simulink model "FDIBenchMark_BLW_66_71"  (Simulink 6.3)
settings: Solver=ode45  StartTime=0.0  StopTime=300  FixedStep=Ts  RelTol=1e-12
InitFcn:
  | FDIBenchMarkData
undefined symbols (not defined in the file or in its folder): a, Addt, Addt2, alpha, alpha_gc, Apb, Apb1, Apb2, Bddt, Bddt2, Bpb, Bpb1, Bpb2, Cddt, Constant_Beta_1_m1, Constant_Beta_3_m1, Constant_Omega_r_m1, Constant_tau_gc, Cpb, Cpb1, Cpb2, Cq, DiscIntNeverNeededParam, eta_gc, Gain_Beta_2_m2, Gain_Omega_r_m2, H, k, K_i, K_opt, K_p, L, m, m_vw, Omega_delta, omega_n, Omega_nom, P_r, R, r, r0, rho, seed, T_sample, Ts, turb_int, turbulence_seeds, u0, xi
libraries: simulink x13
settings Model: Creator=peodg  LastModifiedBy=Administrator  StrictBusMsg=None
settings DebuggingCC: SignalResolutionControl=UseLocalSettings  MultiTaskDSMMsg=error
settings HardwareCC: TargetHWDeviceType=32-bit Generic

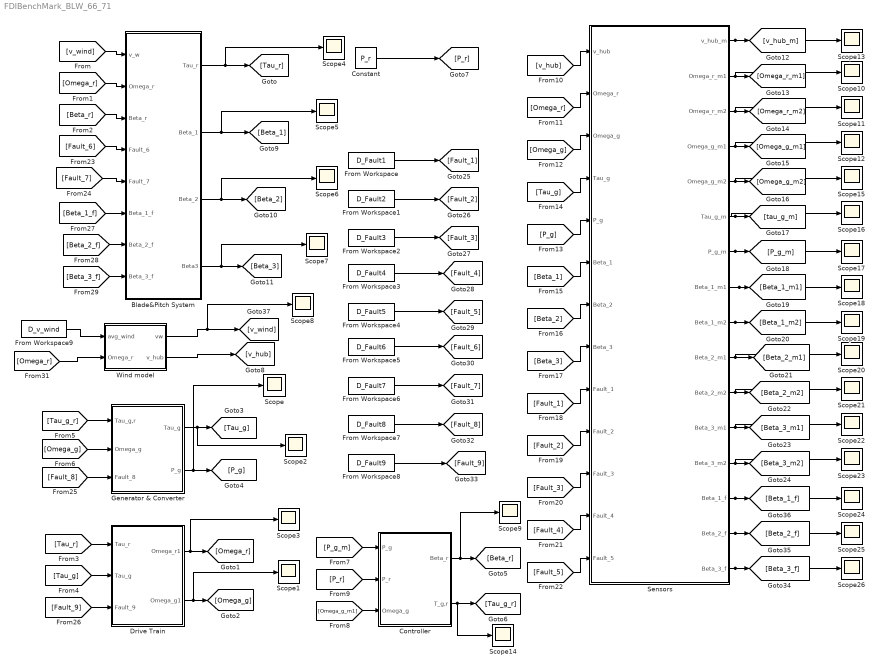
== system FDIBenchMark_BLW_66_71 ==
  Blade&Pitch System : Subsystem
  Constant : Constant  Value=P_r
  Controller : Subsystem
  Drive Train : Subsystem
  From Workspace : FromWorkspace  VariableName=D_Fault1  SampleTime=Ts
  From Workspace1 : FromWorkspace  VariableName=D_Fault2  SampleTime=Ts
  From Workspace2 : FromWorkspace  VariableName=D_Fault3  SampleTime=Ts
  From Workspace3 : FromWorkspace  VariableName=D_Fault4  SampleTime=Ts
  From Workspace4 : FromWorkspace  VariableName=D_Fault5  SampleTime=Ts
  From Workspace5 : FromWorkspace  VariableName=D_Fault6  SampleTime=Ts
  From Workspace6 : FromWorkspace  VariableName=D_Fault7  SampleTime=Ts
  From Workspace7 : FromWorkspace  VariableName=D_Fault8  SampleTime=Ts
  From Workspace8 : FromWorkspace  VariableName=D_Fault9  SampleTime=Ts
  From Workspace9 : FromWorkspace  VariableName=D_v_wind
  Generator & Converter : Subsystem
  Scope{,1..26} (27 alike) : Scope
      Scope settings: YMin=1e+006  YMax=5.25e+006  SaveName=P_g  DataFormat=Array  SampleInput=on  SampleTime=Ts
      Scope1 settings: YMin=64  YMax=66.25  SaveName=Oemga_g1  DataFormat=Array  SampleInput=on  SampleTime=Ts
      Scope10 settings: YMin=1.1  YMax=2.4  SaveName=Omega_r_m1  DataFormat=Array  SampleInput=on  SampleTime=Ts
      Scope11 settings: YMin=-1  YMax=1  SaveName=Omega_r_m2  DataFormat=Array  SampleInput=on  SampleTime=Ts
      Scope12 settings: YMin=-1  YMax=1  SaveName=Omega_g_m1  DataFormat=Array  SampleInput=on  SampleTime=Ts
      Scope13 settings: YMin=-1  YMax=1  SaveName=v_hub_m  DataFormat=Array  SampleInput=on  SampleTime=Ts
      Scope14 settings: YMin=-2.5  YMax=20  SaveName=T_g_r  DataFormat=Array  SampleInput=on  SampleTime=Ts
      Scope15 settings: YMin=-1  YMax=1  SaveName=Omega_g_m2  DataFormat=Array  SampleInput=on  SampleTime=Ts
      Scope16 settings: YMin=-1  YMax=1  SaveName=Tau_g_m  DataFormat=Array  SampleInput=on  SampleTime=Ts
      Scope17 settings: YMin=-1  YMax=1  SaveName=P_g_m  DataFormat=Array  SampleInput=on  SampleTime=Ts
      Scope18 settings: YMin=-1  YMax=1  SaveName=Beta_1_m1  DataFormat=Array  SampleInput=on  SampleTime=Ts
      Scope19 settings: YMin=-1  YMax=1  SaveName=Beta_1_m2  DataFormat=Array  SampleInput=on  SampleTime=Ts
      Scope2 settings: YMin=29400  YMax=29875  SaveName=Tau_g  DataFormat=Array  SampleInput=on  SampleTime=Ts
      Scope20 settings: YMin=-1  YMax=1  SaveName=Beta_2_m1  DataFormat=Array  SampleInput=on  SampleTime=Ts
      Scope21 settings: YMin=-1  YMax=1  SaveName=Beta_2_m2  DataFormat=Array  SampleInput=on  SampleTime=Ts
      Scope22 settings: YMin=-4  YMax=12  SaveName=Beta_3_m1  DataFormat=Array  SampleInput=on  SampleTime=Ts
      Scope23 settings: YMin=-1  YMax=1  SaveName=Beta_3_m2  DataFormat=Array  SampleInput=on  SampleTime=Ts
      Scope24 settings: YMin=-1  YMax=1  SaveName=Beta_1_f  DataFormat=Array  SampleInput=on  SampleTime=Ts
      Scope25 settings: YMin=-1  YMax=1  SaveName=Beta_2_f  DataFormat=Array  SampleInput=on  SampleTime=Ts
      Scope26 settings: YMin=-1  YMax=1  SaveName=Beta_3_f  DataFormat=Array  SampleInput=on  SampleTime=Ts
      Scope3 settings: YMin=0.62  YMax=0.69  SaveName=Omega_r1  DataFormat=Array  SampleInput=on  SampleTime=Ts
      Scope4 settings: YMin=-1e+006  YMax=6e+006  SaveName=Tau_r  DataFormat=Array  SampleInput=on  SampleTime=Ts
      Scope5 settings: YMin=-3  YMax=8  SaveName=Beta1  DataFormat=Array  SampleInput=on  SampleTime=Ts
      Scope6 settings: YMin=-0.3  YMax=0.3  SaveName=Beta  DataFormat=Array  SampleInput=on  SampleTime=Ts
      Scope7 settings: YMin=-2.5  YMax=3.5  SaveName=Beta3  DataFormat=Array  SampleInput=on  SampleTime=Ts
      Scope8 settings: YMin=3  YMax=18  SaveName=Vw  DataFormat=Array  SampleInput=on  SampleTime=Ts
      Scope9 settings: YMin=-2.5  YMax=20  SaveName=Beta_r  DataFormat=Array  SampleInput=on  SampleTime=Ts
  Sensors : Subsystem
  Wind model : Subsystem
  wires:
  [v_wind] -> Blade&Pitch System/1(v_w)
  [Omega_r] -> Blade&Pitch System/2(Omega_r)
  [Beta_r] -> Blade&Pitch System/3(Beta_r)
  [Tau_r] -> Drive Train/1(Tau_r)
  [Tau_g] -> Drive Train/2(Tau_g)
  Drive Train/1(Omega_r1) -> [Omega_r], Scope3/1
  [Tau_g_r] -> Generator & Converter/1(Tau_g,r)
  [Omega_g] -> Generator & Converter/2(Omega_g)
  Generator & Converter/1(Tau_g) -> [Tau_g], Scope2/1
  Generator & Converter/2(P_g) -> [P_g], Scope/1
  [P_g_m] -> Controller/1(P_g)
  [Omega_g_m1] -> Controller/3(Omega_g)
  Controller/1(Beta_r) -> [Beta_r], Scope9/1
  Controller/2(T_g,r) -> [Tau_g_r], Scope14/1
  [P_r] -> Controller/2(P_r)
  Constant/1 -> [P_r]
  Sensors/1(v_hub_m) -> [v_hub_m], Scope13/1
  Sensors/2(Omega_r_m1) -> [Omega_r_m1], Scope10/1
  Sensors/3(Omega_r_m2) -> [Omega_r_m2], Scope11/1
  Sensors/4(Omega_g_m1) -> [Omega_g_m1], Scope12/1
  Sensors/5(Omega_g_m2) -> [Omega_g_m2], Scope15/1
  Sensors/6(Tau_g_m) -> [tau_g_m], Scope16/1
  Sensors/7(P_g_m) -> [P_g_m], Scope17/1
  Sensors/8(Beta_1_m1) -> [Beta_1_m1], Scope18/1
  Sensors/9(Beta_1_m2) -> [Beta_1_m2], Scope19/1
  Sensors/10(Beta_2_m1) -> [Beta_2_m1], Scope20/1
  Sensors/11(Beta_2_m2) -> [Beta_2_m2], Scope21/1
  Sensors/12(Beta_3_m1) -> [Beta_3_m1], Scope22/1
  Sensors/13(Beta_3_m2) -> [Beta_3_m2], Scope23/1
  [v_hub] -> Sensors/1(v_hub)
  [Omega_r] -> Sensors/2(Omega_r)
  [Omega_g] -> Sensors/3(Omega_g)
  [Tau_g] -> Sensors/4(Tau_g)
  [P_g] -> Sensors/5(P_g)
  [Beta_1] -> Sensors/6(Beta_1)
  [Beta_2] -> Sensors/7(Beta_2)
  [Beta_3] -> Sensors/8(Beta_3)
  [Fault_1] -> Sensors/9(Fault_1)
  [Fault_2] -> Sensors/10(Fault_2)
  [Fault_3] -> Sensors/11(Fault_3)
  [Fault_4] -> Sensors/12(Fault_4)
  [Fault_5] -> Sensors/13(Fault_5)
  [Fault_6] -> Blade&Pitch System/4(Fault_6)
  [Fault_7] -> Blade&Pitch System/5(Fault_7)
  [Fault_8] -> Generator & Converter/3(Fault_8)
  [Fault_9] -> Drive Train/3(Fault_9)
  From Workspace8/1 -> [Fault_9]
  From Workspace7/1 -> [Fault_8]
  From Workspace6/1 -> [Fault_7]
  From Workspace5/1 -> [Fault_6]
  From Workspace4/1 -> [Fault_5]
  From Workspace3/1 -> [Fault_4]
  From Workspace2/1 -> [Fault_3]
  From Workspace1/1 -> [Fault_2]
  From Workspace/1 -> [Fault_1]
  Drive Train/2(Omega_g1) -> [Omega_g], Scope1/1
  Sensors/16(Beta_3_f) -> [Beta_3_f], Scope26/1
  Sensors/15(Beta_2_f) -> [Beta_2_f], Scope25/1
  Sensors/14(Beta_1_f) -> [Beta_1_f], Scope24/1
  [Beta_1_f] -> Blade&Pitch System/6(Beta_1_f)
  [Beta_2_f] -> Blade&Pitch System/7(Beta_2_f)
  [Beta_3_f] -> Blade&Pitch System/8(Beta_3_f)
  Blade&Pitch System/4(Beta3) -> [Beta_3], Scope7/1
  Blade&Pitch System/3(Beta_2) -> [Beta_2], Scope6/1
  Blade&Pitch System/2(Beta_1) -> [Beta_1], Scope5/1
  Blade&Pitch System/1(Tau_r) -> [Tau_r], Scope4/1
  Wind model/1(vw) -> [v_wind], Scope8/1
  Wind model/2(v_hub) -> [v_hub]
  [Omega_r] -> Wind model/2(Omega_r)
  From Workspace9/1 -> Wind model/1(avg_wind)

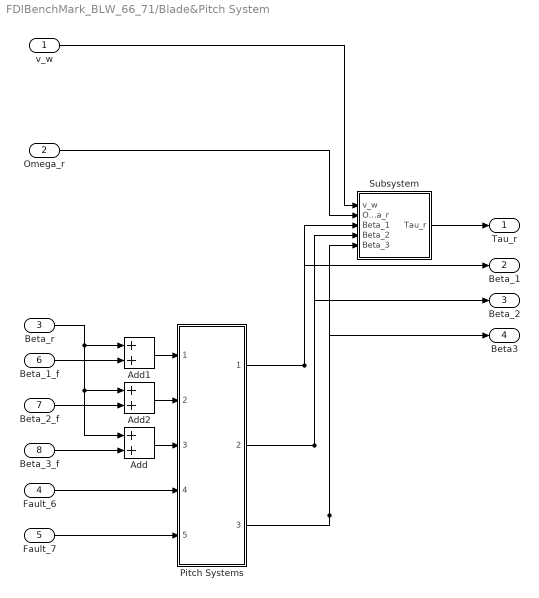
== system FDIBenchMark_BLW_66_71/Blade&Pitch System ==
  v_w : Inport
  Omega_r : Inport  Port=2
  Beta_r : Inport  Port=3
  Fault_6 : Inport  Port=4
  Fault_7 : Inport  Port=5
  Beta_1_f : Inport  Port=6
  Beta_2_f : Inport  Port=7
  Beta_3_f : Inport  Port=8
  Add : Sum  OutScaling=2^-10
  Add1 : Sum  OutScaling=2^-10
  Add2 : Sum  OutScaling=2^-10
  Pitch Systems : Subsystem
  Subsystem : Subsystem
  Tau_r : Outport
  Beta_1 : Outport  Port=2
  Beta_2 : Outport  Port=3
  Beta3 : Outport  Port=4
  wires:
  Pitch Systems/1(Beta_1) -> Subsystem/3(Beta_1), Beta_1/1
  Pitch Systems/2(Beta_2) -> Subsystem/4(Beta_2), Beta_2/1
  Pitch Systems/3(Beta_3) -> Subsystem/5(Beta_3), Beta3/1
  Subsystem/1(Tau_r) -> Tau_r/1
  v_w/1 -> Subsystem/1(v_w)
  Omega_r/1 -> Subsystem/2(Omega_r)
  Fault_6/1 -> Pitch Systems/4(Fault_6)
  Fault_7/1 -> Pitch Systems/5(Fault_7)
  Add/1 -> Pitch Systems/3(Beta_r3)
  Add1/1 -> Pitch Systems/1(Beta_r1)
  Add2/1 -> Pitch Systems/2(Beta_r2)
  Beta_3_f/1 -> Add/2
  Beta_2_f/1 -> Add2/2
  Beta_1_f/1 -> Add1/2
  Beta_r/1 -> Add1/1, Add2/1, Add/1

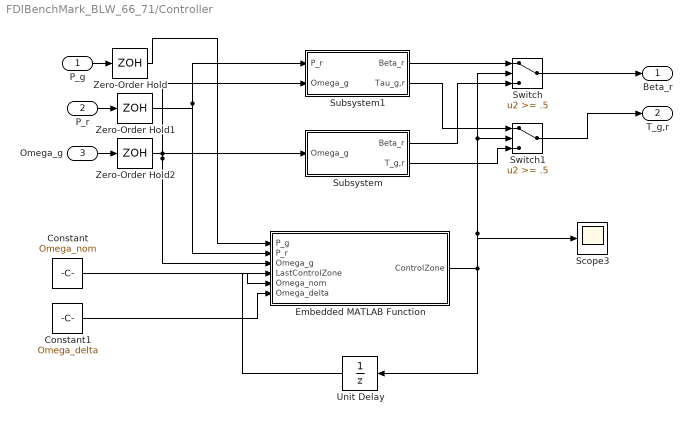
== system FDIBenchMark_BLW_66_71/Controller ==
  P_g : Inport
  P_r : Inport  Port=2
  Omega_g : Inport  Port=3
  Constant : Constant  Value=Omega_nom
  Constant1 : Constant  Value=Omega_delta
  Embedded MATLAB Function : Stateflow chart  TreatAsAtomicUnit=on
      settings: PermitHierarchicalResolution=ParametersOnly
  Scope3 : Scope
      settings: YMin=0.62  YMax=0.69  SaveName=Omega_r  DataFormat=Array  SampleInput=on  SampleTime=Ts
  Subsystem : Subsystem
  Subsystem1 : Subsystem
  Switch : Switch  Threshold=.5
  Switch1 : Switch  Threshold=.5
  Unit Delay : UnitDelay  Orientation=left  SampleTime=Ts
  Zero-Order Hold : ZeroOrderHold  SampleTime=Ts
  Zero-Order Hold1 : ZeroOrderHold  SampleTime=Ts
  Zero-Order Hold2 : ZeroOrderHold  SampleTime=Ts
  Beta_r : Outport
  T_g,r : Outport  Port=2
  wires:
  Embedded MATLAB Function/1(ControlZone) -> Unit Delay/1, Switch/2, Switch1/2, Scope3/1
  Unit Delay/1 -> Embedded MATLAB Function/4(LastControlZone)
  P_g/1 -> Zero-Order Hold/1
  P_r/1 -> Zero-Order Hold1/1
  Omega_g/1 -> Zero-Order Hold2/1
  Switch/1 -> Beta_r/1
  Switch1/1 -> T_g,r/1
  Subsystem1/1(Beta_r) -> Switch/1
  Subsystem/1(Beta_r) -> Switch/3
  Subsystem1/2(Tau_g,r) -> Switch1/1
  Subsystem/2(T_g,r) -> Switch1/3
  Constant/1 -> Embedded MATLAB Function/5(Omega_nom)
  Constant1/1 -> Embedded MATLAB Function/6(Omega_delta)
  Zero-Order Hold/1 -> Embedded MATLAB Function/1(P_g)
  Zero-Order Hold1/1 -> Embedded MATLAB Function/2(P_r), Subsystem1/1(P_r)
  Zero-Order Hold2/1 -> Embedded MATLAB Function/3(Omega_g), Subsystem1/2(Omega_g), Subsystem/1(Omega_g)

== system FDIBenchMark_BLW_66_71/Drive Train ==
  Tau_r : Inport
  Tau_g : Inport  Port=2
  Fault_9 : Inport  Port=3
  Add : Sum  OutScaling=2^-10
  Demux1 : Demux  Outputs=2
  Gain : Gain  Orientation=left  Gain=Addt  Multiplication=Matrix(K*u)
  Gain1 : Gain  Gain=Bddt  Multiplication=Matrix(K*u)
  Gain2 : Gain  Gain=Cddt  Multiplication=Matrix(K*u)
  Gain3 : Gain  Orientation=left  Gain=Addt2  Multiplication=Matrix(K*u)
  Gain4 : Gain  Gain=Bddt2  Multiplication=Matrix(K*u)
  Integrator : Integrator  InitialCondition=[1 100 0]
  Mux : Mux  Inputs=2
  Switch1 : Switch  Threshold=0.5
  Switch2 : Switch  Orientation=left  Threshold=0.5
  Omega_r1 : Outport
  Omega_g1 : Outport  Port=2
  wires:
  Tau_r/1 -> Mux/1
  Tau_g/1 -> Mux/2
  Integrator/1 -> Gain2/1, Gain/1, Gain3/1
  Add/1 -> Integrator/1
  Switch1/1 -> Add/1
  Gain1/1 -> Switch1/1
  Gain4/1 -> Switch1/3
  Gain/1 -> Switch2/1
  Gain3/1 -> Switch2/3
  Switch2/1 -> Add/2
  Demux1/1 -> Omega_r1/1
  Demux1/2 -> Omega_g1/1
  Gain2/1 -> Demux1/1
  Fault_9/1 -> Switch1/2, Switch2/2
  Mux/1 -> Gain1/1, Gain4/1

== system FDIBenchMark_BLW_66_71/Generator & Converter ==
  Tau_g,r : Inport
  Omega_g : Inport  Port=2
  Fault_8 : Inport  Port=3
  Bias : Bias  Bias=Constant_tau_gc
  Divide : Product  Inputs=**  OutScaling=2^-10
  Gain : Gain  Gain=eta_gc
  Switch : Switch  Threshold=0.5
  Transfer Fcn : TransferFcn  Numerator=[alpha_gc]  Denominator=[1 alpha_gc]
  Tau_g : Outport
  P_g : Outport  Port=2
  wires:
  Tau_g,r/1 -> Transfer Fcn/1
  Gain/1 -> P_g/1
  Divide/1 -> Gain/1
  Omega_g/1 -> Divide/2
  Transfer Fcn/1 -> Bias/1, Switch/1
  Fault_8/1 -> Switch/2
  Switch/1 -> Divide/1, Tau_g/1
  Bias/1 -> Switch/3

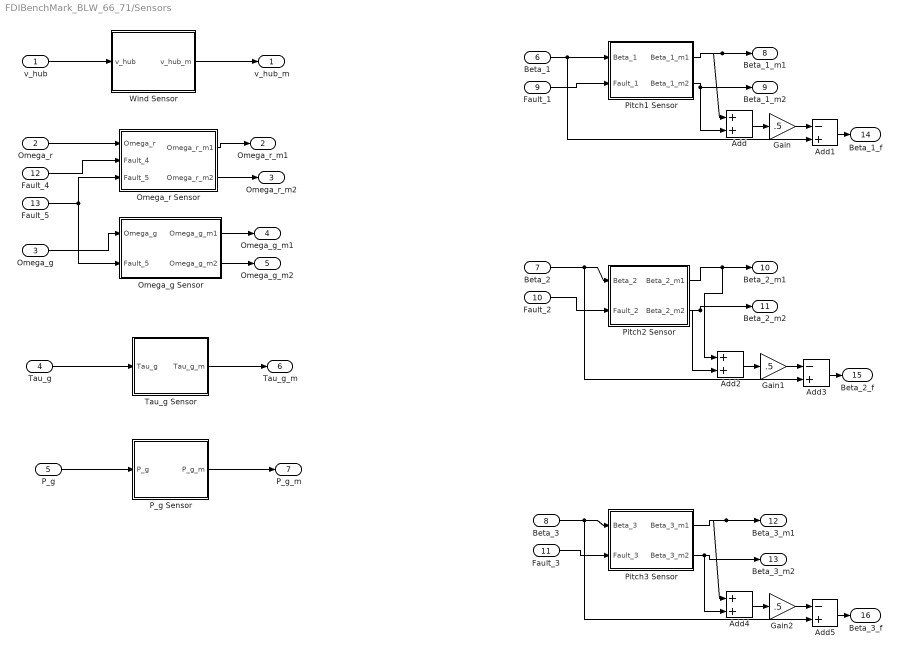
== system FDIBenchMark_BLW_66_71/Sensors ==
  v_hub : Inport
  Omega_r : Inport  Port=2
  Omega_g : Inport  Port=3
  Tau_g : Inport  Port=4
  P_g : Inport  Port=5
  Beta_1 : Inport  Port=6
  Beta_2 : Inport  Port=7
  Beta_3 : Inport  Port=8
  Fault_1 : Inport  Port=9
  Fault_2 : Inport  Port=10
  Fault_3 : Inport  Port=11
  Fault_4 : Inport  Port=12
  Fault_5 : Inport  Port=13
  Add : Sum  OutScaling=2^-10
  Add1 : Sum  Inputs=-+  OutScaling=2^-10
  Add2 : Sum  OutScaling=2^-10
  Add3 : Sum  Inputs=-+  OutScaling=2^-10
  Add4 : Sum  OutScaling=2^-10
  Add5 : Sum  Inputs=-+  OutScaling=2^-10
  Gain : Gain  Gain=.5
  Gain1 : Gain  Gain=.5
  Gain2 : Gain  Gain=.5
  Omega_g Sensor : Subsystem
  Omega_r Sensor : Subsystem
  P_g Sensor : Subsystem
  Pitch1 Sensor : Subsystem
  Pitch2 Sensor : Subsystem
  Pitch3 Sensor : Subsystem
  Tau_g Sensor : Subsystem
  Wind Sensor : Subsystem
  v_hub_m : Outport
  Omega_r_m1 : Outport  Port=2
  Omega_r_m2 : Outport  Port=3
  Omega_g_m1 : Outport  Port=4
  Omega_g_m2 : Outport  Port=5
  Tau_g_m : Outport  Port=6
  P_g_m : Outport  Port=7
  Beta_1_m1 : Outport  Port=8
  Beta_1_m2 : Outport  Port=9
  Beta_2_m1 : Outport  Port=10
  Beta_2_m2 : Outport  Port=11
  Beta_3_m1 : Outport  Port=12
  Beta_3_m2 : Outport  Port=13
  Beta_1_f : Outport  Port=14
  Beta_2_f : Outport  Port=15
  Beta_3_f : Outport  Port=16
  wires:
  Wind Sensor/1(v_hub_m) -> v_hub_m/1
  v_hub/1 -> Wind Sensor/1(v_hub)
  Omega_r/1 -> Omega_r Sensor/1(Omega_r)
  Omega_r Sensor/1(Omega_r_m1) -> Omega_r_m1/1
  Omega_r Sensor/2(Omega_r_m2) -> Omega_r_m2/1
  Omega_g/1 -> Omega_g Sensor/1(Omega_g)
  Omega_g Sensor/1(Omega_g_m1) -> Omega_g_m1/1
  Omega_g Sensor/2(Omega_g_m2) -> Omega_g_m2/1
  Tau_g/1 -> Tau_g Sensor/1(Tau_g)
  Tau_g Sensor/1(Tau_g_m) -> Tau_g_m/1
  P_g/1 -> P_g Sensor/1(P_g)
  P_g Sensor/1(P_g_m) -> P_g_m/1
  Beta_1/1 -> Pitch1 Sensor/1(Beta_1), Add1/2
  Pitch1 Sensor/1(Beta_1_m1) -> Beta_1_m1/1, Add/1
  Pitch1 Sensor/2(Beta_1_m2) -> Beta_1_m2/1, Add/2
  Beta_2/1 -> Pitch2 Sensor/1(Beta_2), Add3/2
  Pitch2 Sensor/1(Beta_2_m1) -> Beta_2_m1/1, Add2/1
  Pitch2 Sensor/2(Beta_2_m2) -> Beta_2_m2/1, Add2/2
  Beta_3/1 -> Pitch3 Sensor/1(Beta_3), Add5/2
  Pitch3 Sensor/1(Beta_3_m1) -> Beta_3_m1/1, Add4/1
  Pitch3 Sensor/2(Beta_3_m2) -> Beta_3_m2/1, Add4/2
  Fault_1/1 -> Pitch1 Sensor/2(Fault_1)
  Fault_2/1 -> Pitch2 Sensor/2(Fault_2)
  Fault_3/1 -> Pitch3 Sensor/2(Fault_3)
  Fault_4/1 -> Omega_r Sensor/2(Fault_4)
  Fault_5/1 -> Omega_r Sensor/3(Fault_5), Omega_g Sensor/2(Fault_5)
  Add/1 -> Gain/1
  Gain/1 -> Add1/1
  Add1/1 -> Beta_1_f/1
  Add2/1 -> Gain1/1
  Gain1/1 -> Add3/1
  Add3/1 -> Beta_2_f/1
  Add4/1 -> Gain2/1
  Gain2/1 -> Add5/1
  Add5/1 -> Beta_3_f/1

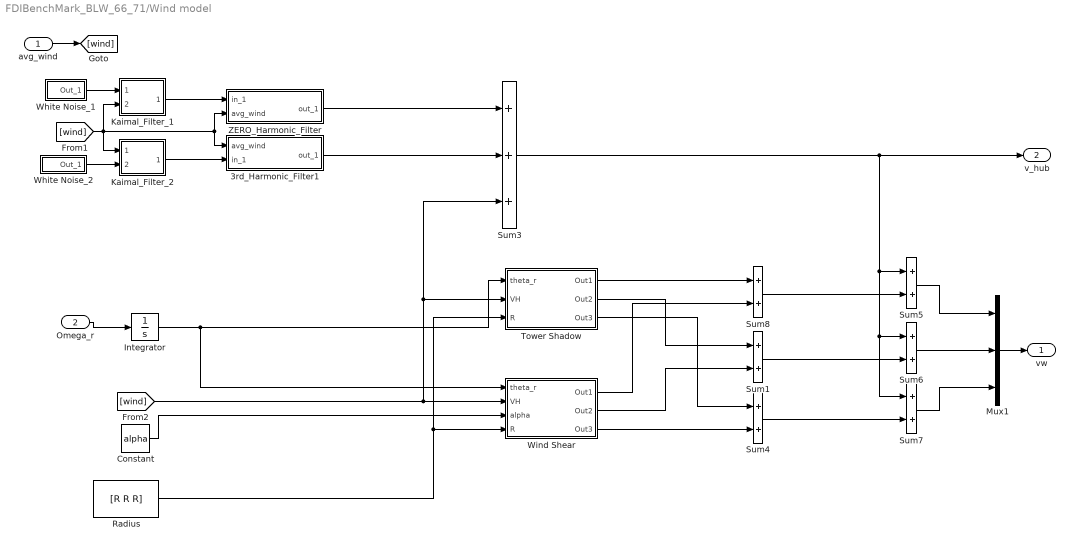
== system FDIBenchMark_BLW_66_71/Wind model ==
  avg_wind : Inport
  Omega_r : Inport  Port=2
  3rd_Harmonic_Filter1 : Subsystem
  Constant : Constant  Value=alpha
  Integrator : Integrator
  Kaimal_Filter_1 : Subsystem
  Kaimal_Filter_2 : Subsystem
  Mux1 : Mux  Inputs=3
  Radius : Constant  Value=[R R R]
  Sum{1,4..8} (6 alike) : Sum  SaturateOnIntegerOverflow=on  InputSameDT=on
  Sum3 : Sum  Inputs=+++  SaturateOnIntegerOverflow=on  InputSameDT=on
  Tower Shadow : Subsystem
  White Noise_1 : Subsystem  mask(Continuous White Noise.){Cov=[1], Ts=T_sample, seed=turbulence_seeds(1)}
      mask prompts: Cov "Noise Power:"; Ts "Sample Time:"
      mask help:
      | White noise for continuous (s-domain) systems.
      | Band-limited using zero-order-hold.
      mask init:
      | r = rand(1,12); r2 = [r(1),r;r,r(12)]; t =[1:13;1:13];
      mask Help: Implemented using white noise into Zero-Order Hold block. The seed and power can be vectors of the same length to produce a vector of white noise sources. For faster simulation, set sample time to the highest value possible but in accordance with the fastest dynamics of system.
      mask Display: plot(t(:),r2(:))
  White Noise_2 : Subsystem  mask(Continuous White Noise.){@1=[1], @2=T_sample, @3=turbulence_seeds(2)}
      mask prompts: @1 "Noise Power:"; @2 "Sample Time:"; @3 "Seed"
      mask help:
      | White noise for continuous (s-domain) systems.
      | Band-limited using zero-order-hold.
      mask init:
      | Cov = @1; Ts = @2; seed = @3; r = rand(1,12); r2 = [r(1),r;r,r(12)]; t =[1:13;1:13];
      mask Help: Implemented using white noise into Zero-Order Hold block. The seed and power can be vectors of the same length to produce a vector of white noise sources. For faster simulation, set sample time to the highest value possible but in accordance with the fastest dynamics of system.
      mask Display: plot(t(:),r2(:))
  Wind Shear : Subsystem
  ZERO_Harmonic_Filter : Subsystem
  vw : Outport  InitialOutput=[u0]
  v_hub : Outport  Port=2  InitialOutput=[u0]
  wires:
  [wind] -> 3rd_Harmonic_Filter1/1(avg_wind), ZERO_Harmonic_Filter/2(avg_wind), Kaimal_Filter_2/1(avg_wind), Kaimal_Filter_1/2(avg_wind)
  avg_wind/1 -> [wind]
  White Noise_2/1(Out_1) -> Kaimal_Filter_2/2(in_1)
  Kaimal_Filter_2/1(out_1) -> 3rd_Harmonic_Filter1/2(in_1)
  Kaimal_Filter_1/1(out_1) -> ZERO_Harmonic_Filter/1(in_1)
  White Noise_1/1(Out_1) -> Kaimal_Filter_1/1(in_1)
  [wind] -> Wind Shear/2(VH), Sum3/3, Tower Shadow/2(VH)
  Constant/1 -> Wind Shear/3(alpha)
  Radius/1 -> Wind Shear/4(R), Tower Shadow/3(R)
  Tower Shadow/1(Out1) -> Sum8/1
  Wind Shear/1(Out1) -> Sum8/2
  Tower Shadow/2(Out2) -> Sum1/1
  Wind Shear/2(Out2) -> Sum1/2
  Tower Shadow/3(Out3) -> Sum4/1
  Wind Shear/3(Out3) -> Sum4/2
  Sum8/1 -> Sum5/2
  Sum1/1 -> Sum6/2
  Sum4/1 -> Sum7/2
  Sum5/1 -> Mux1/1
  Sum6/1 -> Mux1/2
  Sum7/1 -> Mux1/3
  Mux1/1 -> vw/1
  Sum3/1 -> Sum6/1, Sum7/1, Sum5/1, v_hub/1
  3rd_Harmonic_Filter1/1(out_1) -> Sum3/2
  ZERO_Harmonic_Filter/1(out_1) -> Sum3/1
  Omega_r/1 -> Integrator/1
  Integrator/1 -> Tower Shadow/1(theta_r), Wind Shear/1(theta_r)

== system FDIBenchMark_BLW_66_71/Blade&Pitch System/Pitch Systems ==
  Beta_r1 : Inport  OutDataType=fixdt(1,16,0)  OutScaling=[]
  Beta_r2 : Inport  Port=2  OutDataType=fixdt(1,16,0)  OutScaling=[]
  Beta_r3 : Inport  Port=3  OutDataType=fixdt(1,16,0)  OutScaling=[]
  Fault_6 : Inport  Port=4  OutDataType=fixdt(1,16,0)  OutScaling=[]
  Fault_7 : Inport  Port=5  OutDataType=fixdt(1,16,0)  OutScaling=[]
  PitchSystem 1 : Subsystem
  PitchSystem 2 : Subsystem
  PitchSystem 3 : Subsystem
  Beta_1 : Outport  OutDataType=fixdt(1,16,0)  OutScaling=[]
  Beta_2 : Outport  Port=2  OutDataType=fixdt(1,16,0)  OutScaling=[]
  Beta_3 : Outport  Port=3  OutDataType=fixdt(1,16,0)  OutScaling=[]
  wires:
  PitchSystem 1/1(Beta_1) -> Beta_1/1
  PitchSystem 2/1(Beta_2) -> Beta_2/1
  PitchSystem 3/1(Beta_3) -> Beta_3/1
  Fault_7/1 -> PitchSystem 3/2(Fault_7)
  Fault_6/1 -> PitchSystem 2/2(Fault_6)
  Beta_r3/1 -> PitchSystem 3/1(Beta_r)
  Beta_r2/1 -> PitchSystem 2/1(Beta_r)
  Beta_r1/1 -> PitchSystem 1/1(Beta_r)

== system FDIBenchMark_BLW_66_71/Blade&Pitch System/Subsystem ==
  v_w : Inport  OutDataType=fixdt(1,16,0)  OutScaling=[]
  Omega_r : Inport  Port=2  OutDataType=fixdt(1,16,0)  OutScaling=[]
  Beta_1 : Inport  Port=3  OutDataType=fixdt(1,16,0)  OutScaling=[]
  Beta_2 : Inport  Port=4  OutDataType=fixdt(1,16,0)  OutScaling=[]
  Beta_3 : Inport  Port=5  OutDataType=fixdt(1,16,0)  OutScaling=[]
  Add : Sum  Inputs=+++  OutScaling=2^-10
  AeroDyn 1 : Subsystem
  AeroDyn 2 : Subsystem
  AeroDyn 3 : Subsystem
  Demux : Demux  Outputs=3
  Scope1 : Scope
      settings: YMin=0.5225  YMax=0.545  SaveName=ScopeData12
  Scope3 : Scope
      settings: YMin=5  YMax=7.75  SaveName=ScopeData11
  Tau_r : Outport  OutDataType=fixdt(1,16,0)  OutScaling=[]
  wires:
  Omega_r/1 -> AeroDyn 1/2(Omega_r), AeroDyn 3/2(Omega_r), AeroDyn 2/2(Omega_r), Scope1/1
  AeroDyn 1/1(Tau_r1) -> Add/1
  AeroDyn 2/1(Tau_r2) -> Add/2
  AeroDyn 3/1(Tau_r3) -> Add/3
  Beta_1/1 -> AeroDyn 1/3(Beta_1)
  Add/1 -> Tau_r/1
  Beta_2/1 -> AeroDyn 2/3(Beta_2)
  Beta_3/1 -> AeroDyn 3/3(Beta_3)
  v_w/1 -> Demux/1, Scope3/1
  Demux/3 -> AeroDyn 3/1(v_w)
  Demux/2 -> AeroDyn 2/1(v_w)
  Demux/1 -> AeroDyn 1/1(v_w)

== system FDIBenchMark_BLW_66_71/Controller/Subsystem ==
  Omega_g : Inport
  Constant : Constant  Value=0
  Gain : Gain  Gain=K_opt
  Product : Product  RndMeth=Zero
  Beta_r : Outport
  T_g,r : Outport  Port=2
  wires:
  Constant/1 -> Beta_r/1
  Omega_g/1 -> Product/2, Product/1
  Gain/1 -> T_g,r/1
  Product/1 -> Gain/1

== system FDIBenchMark_BLW_66_71/Controller/Subsystem1 ==
  P_r : Inport
  Omega_g : Inport  Port=2
  Add : Sum  OutScaling=2^-10
  Bias : Bias  Bias=-Omega_nom
  Discrete-Time Integrator : DiscreteIntegrator  SampleTime=Ts  LimitOutput=on  UpperSaturationLimit=90  LowerSaturationLimit=-2  ICPrevOutput=DiscIntNeverNeededParam  ICPrevScaledInput=DiscIntNeverNeededParam
  Divide : Product  Inputs=/*  OutScaling=2^-10
  Gain : Gain  Gain=K_p
  Gain1 : Gain  Gain=K_i
  Gain2 : Gain  Gain=1/eta_gc
  Saturation : Saturate  UpperLimit=90  LowerLimit=-2
  Beta_r : Outport
  Tau_g,r : Outport  Port=2
  wires:
  Divide/1 -> Gain2/1
  P_r/1 -> Divide/2
  Omega_g/1 -> Divide/1, Bias/1
  Bias/1 -> Discrete-Time Integrator/1, Gain/1
  Discrete-Time Integrator/1 -> Gain1/1
  Gain1/1 -> Add/2
  Gain/1 -> Add/1
  Add/1 -> Saturation/1
  Saturation/1 -> Beta_r/1
  Gain2/1 -> Tau_g,r/1

== system FDIBenchMark_BLW_66_71/Sensors/Omega_g Sensor ==
  Omega_g : Inport  OutDataType=fixdt(1,16,0)  OutScaling=[]
  Fault_5 : Inport  Port=2  OutDataType=fixdt(1,16,0)  OutScaling=[]
  Add : Sum  OutScaling=2^-10
  Add1 : Sum  OutScaling=2^-10
  Band-Limited White Noise : simulink/Sources/Band-Limited White Noise  Cov=Np_omega_g  Ts=Ts  seed=seed(4)
  Band-Limited White Noise1 : simulink/Sources/Band-Limited White Noise  Cov=Np_omega_g  Ts=Ts  seed=seed(5)
  Gain : Gain  Gain=Gain_Omega_r_m2
  Switch1 : Switch  Threshold=0.5
  Omega_g_m1 : Outport  OutDataType=fixdt(1,16,0)  OutScaling=[]
  Omega_g_m2 : Outport  Port=2  OutDataType=fixdt(1,16,0)  OutScaling=[]
  wires:
  Band-Limited White Noise1/1 -> Add1/2
  Band-Limited White Noise/1 -> Add/1
  Omega_g/1 -> Add1/1, Add/2
  Add/1 -> Omega_g_m1/1
  Add1/1 -> Switch1/1, Gain/1
  Switch1/1 -> Omega_g_m2/1
  Fault_5/1 -> Switch1/2
  Gain/1 -> Switch1/3

== system FDIBenchMark_BLW_66_71/Sensors/Omega_r Sensor ==
  Omega_r : Inport  OutDataType=fixdt(1,16,0)  OutScaling=[]
  Fault_4 : Inport  Port=2  OutDataType=fixdt(1,16,0)  OutScaling=[]
  Fault_5 : Inport  Port=3  OutDataType=fixdt(1,16,0)  OutScaling=[]
  Add : Sum  OutScaling=2^-10
  Add1 : Sum  OutScaling=2^-10
  Band-Limited White Noise : simulink/Sources/Band-Limited White Noise  Cov=Np_omega_r  Ts=Ts  seed=seed(2)
  Band-Limited White Noise1 : simulink/Sources/Band-Limited White Noise  Cov=Np_omega_r  Ts=Ts  seed=seed(3)
  Constant : Constant  Value=Constant_Omega_r_m1
  Gain : Gain  Gain=Gain_Omega_r_m2
  Switch : Switch  Threshold=0.5
  Switch1 : Switch  Threshold=0.5
  Omega_r_m1 : Outport  OutDataType=fixdt(1,16,0)  OutScaling=[]
  Omega_r_m2 : Outport  Port=2  OutDataType=fixdt(1,16,0)  OutScaling=[]
  wires:
  Omega_r/1 -> Add/2, Add1/1
  Band-Limited White Noise/1 -> Add/1
  Band-Limited White Noise1/1 -> Add1/2
  Fault_4/1 -> Switch/2
  Constant/1 -> Switch/3
  Add/1 -> Switch/1
  Switch/1 -> Omega_r_m1/1
  Add1/1 -> Switch1/1, Gain/1
  Switch1/1 -> Omega_r_m2/1
  Fault_5/1 -> Switch1/2
  Gain/1 -> Switch1/3

== system FDIBenchMark_BLW_66_71/Sensors/P_g Sensor ==
  P_g : Inport  OutDataType=fixdt(1,16,0)  OutScaling=[]
  Add : Sum  OutScaling=2^-10
  Band-Limited White Noise : simulink/Sources/Band-Limited White Noise  Cov=Np_P_g  Ts=Ts  seed=seed(7)
  P_g_m : Outport  OutDataType=fixdt(1,16,0)  OutScaling=[]
  wires:
  Band-Limited White Noise/1 -> Add/2
  P_g/1 -> Add/1
  Add/1 -> P_g_m/1

== system FDIBenchMark_BLW_66_71/Sensors/Pitch1 Sensor ==
  Beta_1 : Inport  OutDataType=fixdt(1,16,0)  OutScaling=[]
  Fault_1 : Inport  Port=2  OutDataType=fixdt(1,16,0)  OutScaling=[]
  Add : Sum  OutScaling=2^-10
  Add1 : Sum  OutScaling=2^-10
  Band-Limited White Noise : simulink/Sources/Band-Limited White Noise  Cov=Np_beta  Ts=Ts  seed=seed(8)
  Band-Limited White Noise1 : simulink/Sources/Band-Limited White Noise  Cov=Np_beta  Ts=Ts  seed=seed(9)
  Constant : Constant  Value=Constant_Beta_1_m1
  Switch : Switch  Threshold=0.5
  Beta_1_m1 : Outport  OutDataType=fixdt(1,16,0)  OutScaling=[]
  Beta_1_m2 : Outport  Port=2  OutDataType=fixdt(1,16,0)  OutScaling=[]
  wires:
  Band-Limited White Noise1/1 -> Add1/2
  Add1/1 -> Beta_1_m2/1
  Band-Limited White Noise/1 -> Add/1
  Beta_1/1 -> Add1/1, Add/2
  Fault_1/1 -> Switch/2
  Constant/1 -> Switch/3
  Add/1 -> Switch/1
  Switch/1 -> Beta_1_m1/1

== system FDIBenchMark_BLW_66_71/Sensors/Pitch2 Sensor ==
  Beta_2 : Inport  OutDataType=fixdt(1,16,0)  OutScaling=[]
  Fault_2 : Inport  Port=2  OutDataType=fixdt(1,16,0)  OutScaling=[]
  Add : Sum  OutScaling=2^-10
  Add1 : Sum  OutScaling=2^-10
  Band-Limited White Noise : simulink/Sources/Band-Limited White Noise  Cov=Np_beta  Ts=Ts  seed=seed(10)
  Band-Limited White Noise1 : simulink/Sources/Band-Limited White Noise  Cov=Np_beta  Ts=Ts  seed=seed(11)
  Gain : Gain  Gain=Gain_Beta_2_m2
  Switch : Switch  Threshold=.5
  Beta_2_m1 : Outport  OutDataType=fixdt(1,16,0)  OutScaling=[]
  Beta_2_m2 : Outport  Port=2  OutDataType=fixdt(1,16,0)  OutScaling=[]
  wires:
  Band-Limited White Noise1/1 -> Add1/2
  Band-Limited White Noise/1 -> Add/1
  Beta_2/1 -> Add1/1, Add/2
  Add/1 -> Beta_2_m1/1
  Add1/1 -> Switch/1, Gain/1
  Gain/1 -> Switch/3
  Switch/1 -> Beta_2_m2/1
  Fault_2/1 -> Switch/2

== system FDIBenchMark_BLW_66_71/Sensors/Pitch3 Sensor ==
  Beta_3 : Inport  OutDataType=fixdt(1,16,0)  OutScaling=[]
  Fault_3 : Inport  Port=2  OutDataType=fixdt(1,16,0)  OutScaling=[]
  Add : Sum  OutScaling=2^-10
  Add1 : Sum  OutScaling=2^-10
  Band-Limited White Noise1 : simulink/Sources/Band-Limited White Noise  Cov=Np_beta  Ts=Ts  seed=seed(13)
  Band-Limited White Noise2 : simulink/Sources/Band-Limited White Noise  Cov=Np_beta  Ts=Ts  seed=seed(12)
  Constant : Constant  Value=Constant_Beta_3_m1
  Switch : Switch  Threshold=0.5
  Beta_3_m1 : Outport  OutDataType=fixdt(1,16,0)  OutScaling=[]
  Beta_3_m2 : Outport  Port=2  OutDataType=fixdt(1,16,0)  OutScaling=[]
  wires:
  Band-Limited White Noise1/1 -> Add1/2
  Add1/1 -> Beta_3_m2/1
  Band-Limited White Noise2/1 -> Add/1
  Beta_3/1 -> Add1/1, Add/2
  Fault_3/1 -> Switch/2
  Constant/1 -> Switch/3
  Add/1 -> Switch/1
  Switch/1 -> Beta_3_m1/1

== system FDIBenchMark_BLW_66_71/Sensors/Tau_g Sensor ==
  Tau_g : Inport  OutDataType=fixdt(1,16,0)  OutScaling=[]
  Add : Sum  OutScaling=2^-10
  Band-Limited White Noise : simulink/Sources/Band-Limited White Noise  Cov=Np_tau_g  Ts=Ts  seed=seed(6)
  Tau_g_m : Outport  OutDataType=fixdt(1,16,0)  OutScaling=[]
  wires:
  Add/1 -> Tau_g_m/1
  Tau_g/1 -> Add/1
  Band-Limited White Noise/1 -> Add/2

== system FDIBenchMark_BLW_66_71/Sensors/Wind Sensor ==
  v_hub : Inport  OutDataType=fixdt(1,16,0)  OutScaling=[]
  Add : Sum  Inputs=+++  OutScaling=2^-10
  Band-Limited White Noise : simulink/Sources/Band-Limited White Noise  Cov=Np_vm  Ts=Ts  seed=seed(1)
  Constant : Constant  Value=m_vw
  v_hub_m : Outport  OutDataType=fixdt(1,16,0)  OutScaling=[]
  wires:
  v_hub/1 -> Add/1
  Add/1 -> v_hub_m/1
  Constant/1 -> Add/3
  Band-Limited White Noise/1 -> Add/2

== system FDIBenchMark_BLW_66_71/Wind model/3rd_Harmonic_Filter1 ==
  avg_wind : Inport
  in_1 : Inport  Port=2
  3rd harmonic Filter : Subsystem
  Unit Delay : UnitDelay  SampleTime=T_sample
  out_1 : Outport
  wires:
  3rd harmonic Filter/1(Out) -> out_1/1
  avg_wind/1 -> 3rd harmonic Filter/1(avg_wind)
  in_1/1 -> Unit Delay/1
  Unit Delay/1 -> 3rd harmonic Filter/2(In)

== system FDIBenchMark_BLW_66_71/Wind model/Kaimal_Filter_1 ==
  in_1 : Inport
  avg_wind : Inport  Port=2
  Fcn : Fcn  Expr=turb_int*sqrt(L*u(1))/100/sqrt(2)
  Kaimal Filter : Subsystem
  Product : Product  SaturateOnIntegerOverflow=on
  Unit Delay : UnitDelay  SampleTime=T_sample
  out_1 : Outport
  wires:
  Product/1 -> out_1/1
  Kaimal Filter/1(Out) -> Product/2
  Fcn/1 -> Product/1
  avg_wind/1 -> Fcn/1, Kaimal Filter/1(avg_wind)
  in_1/1 -> Unit Delay/1
  Unit Delay/1 -> Kaimal Filter/2(In)

== system FDIBenchMark_BLW_66_71/Wind model/Kaimal_Filter_2 ==
  avg_wind : Inport
  in_1 : Inport  Port=2
  Fcn : Fcn  Expr=turb_int*sqrt(L*u(1))/100/sqrt(2)
  Kaimal Filter : Subsystem
  Product : Product  SaturateOnIntegerOverflow=on
  Unit Delay : UnitDelay  SampleTime=T_sample
  out_1 : Outport
  wires:
  Unit Delay/1 -> Kaimal Filter/2(In)
  in_1/1 -> Unit Delay/1
  avg_wind/1 -> Kaimal Filter/1(avg_wind), Fcn/1
  Fcn/1 -> Product/1
  Kaimal Filter/1(Out) -> Product/2
  Product/1 -> out_1/1

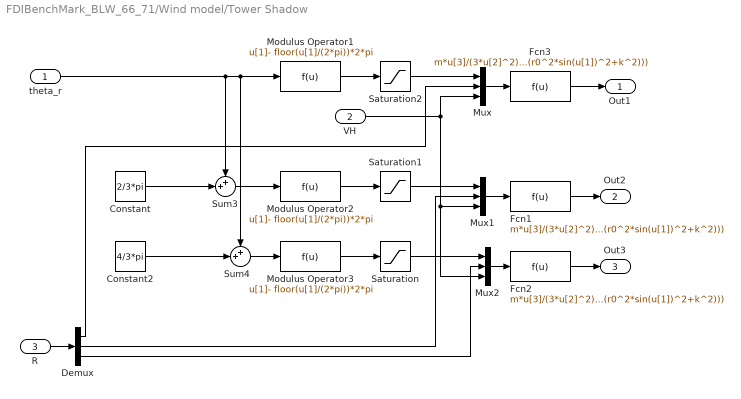
== system FDIBenchMark_BLW_66_71/Wind model/Tower Shadow ==
  theta_r : Inport
  VH : Inport  Port=2
  R : Inport  Port=3
  Constant : Constant  Value=2/3*pi
  Constant2 : Constant  Value=4/3*pi
  Demux : Demux  Outputs=3
  Fcn1 : Fcn  Expr=m*u[3]/(3*u[2]^2)*(a^2*2*(u[2]^2-r0^2)/((u[2]^2+r0^2)*sin(u[1])^2+2*k^2)+2*a^2*k^2*(r0^2-u[2]^2)/((u[2]^2*sin(u[1])^2+k^2)*(r0^2*sin(u[1])^2+k^2)))
  Fcn2 : Fcn  Expr=m*u[3]/(3*u[2]^2)*(a^2*2*(u[2]^2-r0^2)/((u[2]^2+r0^2)*sin(u[1])^2+2*k^2)+2*a^2*k^2*(r0^2-u[2]^2)/((u[2]^2*sin(u[1])^2+k^2)*(r0^2*sin(u[1])^2+k^2)))
  Fcn3 : Fcn  Expr=m*u[3]/(3*u[2]^2)*(a^2*2*(u[2]^2-r0^2)/((u[2]^2+r0^2)*sin(u[1])^2+2*k^2)+2*a^2*k^2*(r0^2-u[2]^2)/((u[2]^2*sin(u[1])^2+k^2)*(r0^2*sin(u[1])^2+k^2)))
  Modulus Operator1 : Fcn  Expr=u[1]- floor(u[1]/(2*pi))*2*pi
  Modulus Operator2 : Fcn  Expr=u[1]- floor(u[1]/(2*pi))*2*pi
  Modulus Operator3 : Fcn  Expr=u[1]- floor(u[1]/(2*pi))*2*pi
  Mux : Mux  Inputs=3
  Mux1 : Mux  Inputs=3
  Mux2 : Mux  Inputs=3
  Saturation : Saturate  UpperLimit=3*pi/2  LowerLimit=pi/2
  Saturation1 : Saturate  UpperLimit=3*pi/2  LowerLimit=pi/2
  Saturation2 : Saturate  UpperLimit=3*pi/2  LowerLimit=pi/2
  Sum3 : Sum  Inputs=++|
  Sum4 : Sum  Inputs=++|
  Out1 : Outport  OutDataType=fixdt(1,16,0)  OutScaling=[]
  Out2 : Outport  Port=2  OutDataType=fixdt(1,16,0)  OutScaling=[]
  Out3 : Outport  Port=3  OutDataType=fixdt(1,16,0)  OutScaling=[]
  wires:
  theta_r/1 -> Sum3/1, Sum4/1, Modulus Operator1/1
  Sum4/1 -> Modulus Operator3/1
  Constant2/1 -> Sum4/2
  Sum3/1 -> Modulus Operator2/1
  Constant/1 -> Sum3/2
  Modulus Operator1/1 -> Saturation2/1
  Modulus Operator2/1 -> Saturation1/1
  Modulus Operator3/1 -> Saturation/1
  Mux/1 -> Fcn3/1
  Saturation2/1 -> Mux/1
  Demux/1 -> Mux/2
  R/1 -> Demux/1
  Mux1/1 -> Fcn1/1
  Saturation1/1 -> Mux1/1
  Demux/2 -> Mux1/2
  Mux2/1 -> Fcn2/1
  Saturation/1 -> Mux2/1
  Demux/3 -> Mux2/2
  VH/1 -> Mux/3, Mux2/3, Mux1/3
  Fcn3/1 -> Out1/1
  Fcn1/1 -> Out2/1
  Fcn2/1 -> Out3/1

== system FDIBenchMark_BLW_66_71/Wind model/White Noise_1 ==
  Gain : Gain  Gain=[sqrt(Cov)]/[sqrt(Ts)]  SaturateOnIntegerOverflow=on
  White Noise : RandomNumber  Seed=seed  SampleTime=Ts
  Zero-Order Hold : ZeroOrderHold  SampleTime=Ts
  Out_1 : Outport
  wires:
  White Noise/1 -> Zero-Order Hold/1
  Gain/1 -> Out_1/1
  Zero-Order Hold/1 -> Gain/1

== system FDIBenchMark_BLW_66_71/Wind model/White Noise_2 ==
  Gain : Gain  Gain=[sqrt(Cov)]/[sqrt(Ts)]  SaturateOnIntegerOverflow=on
  White Noise : RandomNumber  Seed=seed  SampleTime=Ts
  Zero-Order Hold : ZeroOrderHold  SampleTime=Ts
  Out_1 : Outport
  wires:
  White Noise/1 -> Zero-Order Hold/1
  Gain/1 -> Out_1/1
  Zero-Order Hold/1 -> Gain/1

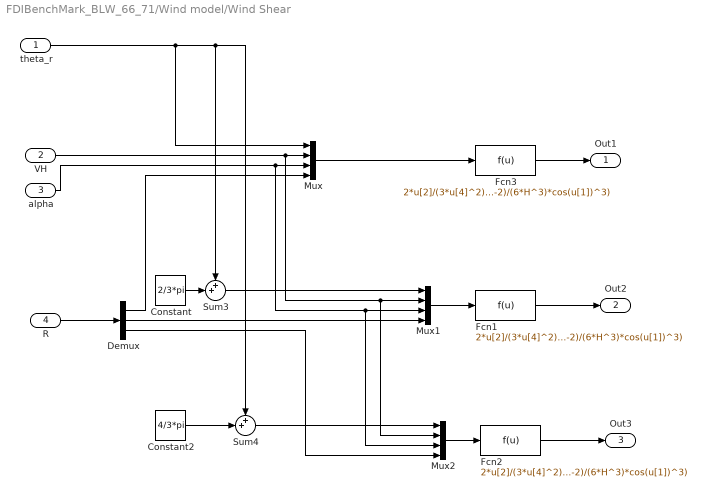
== system FDIBenchMark_BLW_66_71/Wind model/Wind Shear ==
  theta_r : Inport
  VH : Inport  Port=2
  alpha : Inport  Port=3
  R : Inport  Port=4
  Constant : Constant  Value=2/3*pi
  Constant2 : Constant  Value=4/3*pi
  Demux : Demux  Outputs=3
  Fcn1 : Fcn  Expr=2*u[2]/(3*u[4]^2)*(u[4]^3/3*u[3]/H*cos(u[1])+u[4]^4/4*u[3]*(u[3]-1)/(2*H^2)*cos(u[1])^2+u[4]^5/5*u[3]*(u[3]-1)*(u[3]-2)/(6*H^3)*cos(u[1])^3)
  Fcn2 : Fcn  Expr=2*u[2]/(3*u[4]^2)*(u[4]^3/3*u[3]/H*cos(u[1])+u[4]^4/4*u[3]*(u[3]-1)/(2*H^2)*cos(u[1])^2+u[4]^5/5*u[3]*(u[3]-1)*(u[3]-2)/(6*H^3)*cos(u[1])^3)
  Fcn3 : Fcn  Expr=2*u[2]/(3*u[4]^2)*(u[4]^3/3*u[3]/H*cos(u[1])+u[4]^4/4*u[3]*(u[3]-1)/(2*H^2)*cos(u[1])^2+u[4]^5/5*u[3]*(u[3]-1)*(u[3]-2)/(6*H^3)*cos(u[1])^3)
  Mux : Mux
  Mux1 : Mux
  Mux2 : Mux
  Sum3 : Sum  Inputs=++|
  Sum4 : Sum  Inputs=++|
  Out1 : Outport  OutDataType=fixdt(1,16,0)  OutScaling=[]
  Out2 : Outport  Port=2  OutDataType=fixdt(1,16,0)  OutScaling=[]
  Out3 : Outport  Port=3  OutDataType=fixdt(1,16,0)  OutScaling=[]
  wires:
  theta_r/1 -> Sum3/1, Sum4/1, Mux/1
  VH/1 -> Mux/2, Mux1/2, Mux2/2
  Sum4/1 -> Mux2/1
  Constant2/1 -> Sum4/2
  Sum3/1 -> Mux1/1
  Constant/1 -> Sum3/2
  alpha/1 -> Mux/3, Mux1/3, Mux2/3
  Fcn2/1 -> Out3/1
  Fcn1/1 -> Out2/1
  Mux/1 -> Fcn3/1
  R/1 -> Demux/1
  Demux/1 -> Mux/4
  Mux1/1 -> Fcn1/1
  Mux2/1 -> Fcn2/1
  Demux/2 -> Mux1/4
  Demux/3 -> Mux2/4
  Fcn3/1 -> Out1/1

== system FDIBenchMark_BLW_66_71/Wind model/ZERO_Harmonic_Filter ==
  in_1 : Inport
  avg_wind : Inport  Port=2
  Unit Delay : UnitDelay  SampleTime=T_sample
  ZERO harmonic Filter : Subsystem
  out_1 : Outport
  wires:
  Unit Delay/1 -> ZERO harmonic Filter/2(In)
  in_1/1 -> Unit Delay/1
  avg_wind/1 -> ZERO harmonic Filter/1(avg_wind)
  ZERO harmonic Filter/1(Out) -> out_1/1

== system FDIBenchMark_BLW_66_71/Blade&Pitch System/Pitch Systems/PitchSystem 1 ==
  Beta_r : Inport
  Transfer Fcn : TransferFcn  Numerator=[omega_n^2]  Denominator=[1 2*xi*omega_n omega_n^2]
  Beta_1 : Outport
  wires:
  Beta_r/1 -> Transfer Fcn/1
  Transfer Fcn/1 -> Beta_1/1

== system FDIBenchMark_BLW_66_71/Blade&Pitch System/Pitch Systems/PitchSystem 2 ==
  Beta_r : Inport
  Fault_6 : Inport  Port=2
  Add : Sum  OutScaling=2^-10
  Gain : Gain  Orientation=left  Gain=Apb  Multiplication=Matrix(K*u)
  Gain1 : Gain  Gain=Bpb  Multiplication=Matrix(K*u)
  Gain2 : Gain  Gain=Cpb  Multiplication=Matrix(K*u)
  Gain3 : Gain  Orientation=left  Gain=Apb1  Multiplication=Matrix(K*u)
  Gain4 : Gain  Gain=Bpb1  Multiplication=Matrix(K*u)
  Gain5 : Gain  Gain=Cpb1  Multiplication=Matrix(K*u)
  Integrator : Integrator
  Switch1 : Switch  Threshold=0.5
  Switch2 : Switch  Orientation=left  Threshold=0.5
  Switch3 : Switch  Threshold=0.5
  Beta_2 : Outport
  wires:
  Integrator/1 -> Gain/1, Gain3/1, Gain2/1, Gain5/1
  Add/1 -> Integrator/1
  Switch1/1 -> Add/1
  Gain1/1 -> Switch1/1
  Gain4/1 -> Switch1/3
  Gain/1 -> Switch2/1
  Gain3/1 -> Switch2/3
  Switch2/1 -> Add/2
  Fault_6/1 -> Switch1/2, Switch2/2, Switch3/2
  Beta_r/1 -> Gain1/1, Gain4/1
  Gain2/1 -> Switch3/1
  Switch3/1 -> Beta_2/1
  Gain5/1 -> Switch3/3

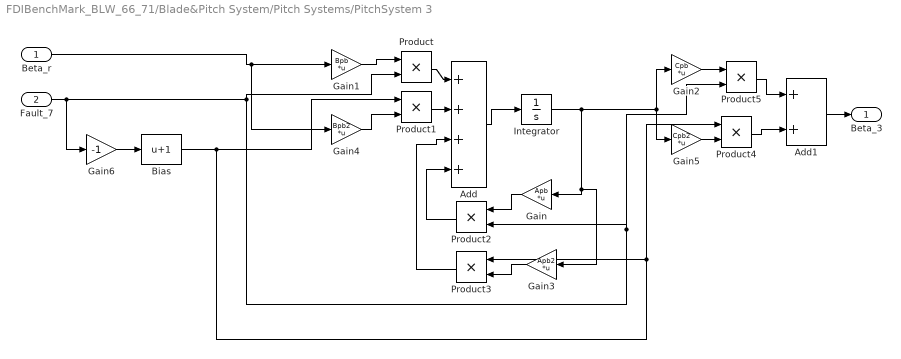
== system FDIBenchMark_BLW_66_71/Blade&Pitch System/Pitch Systems/PitchSystem 3 ==
  Beta_r : Inport
  Fault_7 : Inport  Port=2
  Add : Sum  Inputs=++++  OutScaling=2^-10
  Add1 : Sum  OutScaling=2^-10
  Bias : Bias  Bias=1
  Gain : Gain  Orientation=left  Gain=Apb  Multiplication=Matrix(K*u)
  Gain1 : Gain  Gain=Bpb  Multiplication=Matrix(K*u)
  Gain2 : Gain  Gain=Cpb  Multiplication=Matrix(K*u)
  Gain3 : Gain  Orientation=left  Gain=Apb2  Multiplication=Matrix(K*u)
  Gain4 : Gain  Gain=Bpb2  Multiplication=Matrix(K*u)
  Gain5 : Gain  Gain=Cpb2  Multiplication=Matrix(K*u)
  Gain6 : Gain  Gain=-1
  Integrator : Integrator
  Product{,1,4..5} (4 alike) : Product  RndMeth=Zero
  Product2 : Product  Orientation=left  RndMeth=Zero
  Product3 : Product  Orientation=left  RndMeth=Zero
  Beta_3 : Outport
  wires:
  Beta_r/1 -> Gain4/1, Gain1/1
  Fault_7/1 -> Product2/2, Product5/2, Product/2, Gain6/1
  Gain4/1 -> Product1/2
  Add/1 -> Integrator/1
  Integrator/1 -> Gain5/1, Gain2/1, Gain3/1, Gain/1
  Product/1 -> Add/1
  Gain1/1 -> Product/1
  Product1/1 -> Add/2
  Gain3/1 -> Product3/2
  Gain/1 -> Product2/1
  Product2/1 -> Add/4
  Product3/1 -> Add/3
  Add1/1 -> Beta_3/1
  Gain2/1 -> Product5/1
  Gain5/1 -> Product4/2
  Product4/1 -> Add1/2
  Product5/1 -> Add1/1
  Gain6/1 -> Bias/1
  Bias/1 -> Product1/1, Product3/1, Product4/1

== system FDIBenchMark_BLW_66_71/Blade&Pitch System/Subsystem/AeroDyn 1 ==
  v_w : Inport  Orientation=down  OutDataType=fixdt(1,16,0)  OutScaling=[]
  Omega_r : Inport  Port=2  OutDataType=fixdt(1,16,0)  OutScaling=[]
  Beta_1 : Inport  Port=3  OutDataType=fixdt(1,16,0)  OutScaling=[]
  Divide : Product  Inputs=/*  OutScaling=2^-10
  Divide1 : Product  Inputs=***  OutScaling=2^-10
  Gain : Gain  Gain=R
  Gain1 : Gain  Gain=rho*pi*R^3/6
  Lookup Table (2-D) : Lookup2D  RowIndex=Lambda  ColumnIndex=Angle  OutputValues=Cq
  Tau_r1 : Outport  OutDataType=fixdt(1,16,0)  OutScaling=[]
  wires:
  Divide/1 -> Lookup Table (2-D)/1
  Gain/1 -> Divide/2
  v_w/1 -> Divide/1, Divide1/2, Divide1/1
  Lookup Table (2-D)/1 -> Divide1/3
  Divide1/1 -> Gain1/1
  Omega_r/1 -> Gain/1
  Gain1/1 -> Tau_r1/1
  Beta_1/1 -> Lookup Table (2-D)/2

== system FDIBenchMark_BLW_66_71/Blade&Pitch System/Subsystem/AeroDyn 2 ==
  v_w : Inport  Orientation=down  OutDataType=fixdt(1,16,0)  OutScaling=[]
  Omega_r : Inport  Port=2  OutDataType=fixdt(1,16,0)  OutScaling=[]
  Beta_2 : Inport  Port=3  OutDataType=fixdt(1,16,0)  OutScaling=[]
  Divide : Product  Inputs=/*  OutScaling=2^-10
  Divide1 : Product  Inputs=***  OutScaling=2^-10
  Gain : Gain  Gain=R
  Gain1 : Gain  Gain=rho*pi*R^3/6
  Lookup Table (2-D) : Lookup2D  RowIndex=Lambda  ColumnIndex=Angle  OutputValues=Cq
  Tau_r2 : Outport  OutDataType=fixdt(1,16,0)  OutScaling=[]
  wires:
  Beta_2/1 -> Lookup Table (2-D)/2
  Gain1/1 -> Tau_r2/1
  Omega_r/1 -> Gain/1
  Divide1/1 -> Gain1/1
  Lookup Table (2-D)/1 -> Divide1/3
  v_w/1 -> Divide1/1, Divide1/2, Divide/1
  Gain/1 -> Divide/2
  Divide/1 -> Lookup Table (2-D)/1

== system FDIBenchMark_BLW_66_71/Blade&Pitch System/Subsystem/AeroDyn 3 ==
  v_w : Inport  Orientation=down  OutDataType=fixdt(1,16,0)  OutScaling=[]
  Omega_r : Inport  Port=2  OutDataType=fixdt(1,16,0)  OutScaling=[]
  Beta_3 : Inport  Port=3  OutDataType=fixdt(1,16,0)  OutScaling=[]
  Divide : Product  Inputs=/*  OutScaling=2^-10
  Divide1 : Product  Inputs=***  OutScaling=2^-10
  Gain : Gain  Gain=R
  Gain1 : Gain  Gain=rho*pi*R^3/6
  Lookup Table (2-D) : Lookup2D  RowIndex=Lambda  ColumnIndex=Angle  OutputValues=Cq
  Tau_r3 : Outport  OutDataType=fixdt(1,16,0)  OutScaling=[]
  wires:
  Divide/1 -> Lookup Table (2-D)/1
  Gain/1 -> Divide/2
  v_w/1 -> Divide/1, Divide1/2, Divide1/1
  Lookup Table (2-D)/1 -> Divide1/3
  Divide1/1 -> Gain1/1
  Omega_r/1 -> Gain/1
  Gain1/1 -> Tau_r3/1
  Beta_3/1 -> Lookup Table (2-D)/2

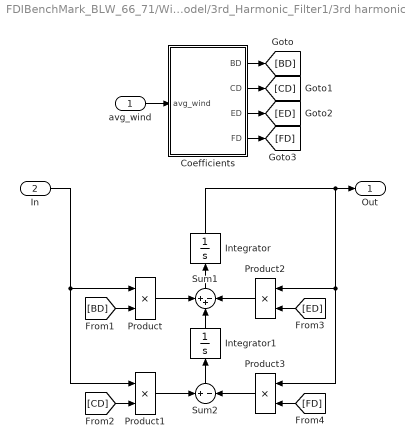
== system FDIBenchMark_BLW_66_71/Wind model/3rd_Harmonic_Filter1/3rd harmonic Filter ==
  avg_wind : Inport
  In : Inport  Port=2
  Coefficients : Subsystem
  Integrator : Integrator  Orientation=up
  Integrator1 : Integrator  Orientation=up
  Product : Product  SaturateOnIntegerOverflow=on
  Product1 : Product  SaturateOnIntegerOverflow=on
  Product2 : Product  Orientation=left  SaturateOnIntegerOverflow=on
  Product3 : Product  Orientation=left  SaturateOnIntegerOverflow=on
  Sum1 : Sum  Orientation=up  Inputs=++-  SaturateOnIntegerOverflow=on
  Sum2 : Sum  Orientation=up  Inputs=+|-  SaturateOnIntegerOverflow=on
  Out : Outport
  wires:
  avg_wind/1 -> Coefficients/1(avg_wind)
  Coefficients/4(FD) -> [FD]
  Coefficients/3(ED) -> [ED]
  Coefficients/2(CD) -> [CD]
  Coefficients/1(BD) -> [BD]
  [FD] -> Product3/2
  [ED] -> Product2/2
  [CD] -> Product1/2
  [BD] -> Product/2
  In/1 -> Product1/1, Product/1
  Product1/1 -> Sum2/1
  Product3/1 -> Sum2/2
  Sum2/1 -> Integrator1/1
  Product2/1 -> Sum1/3
  Integrator1/1 -> Sum1/2
  Product/1 -> Sum1/1
  Sum1/1 -> Integrator/1
  Integrator/1 -> Out/1, Product3/1, Product2/1

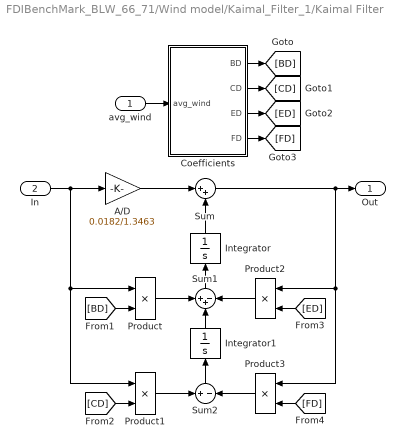
== system FDIBenchMark_BLW_66_71/Wind model/Kaimal_Filter_1/Kaimal Filter ==
  avg_wind : Inport
  In : Inport  Port=2
  A/D : Gain  Gain=0.0182/1.3463  SaturateOnIntegerOverflow=on
  Coefficients : Subsystem
  Integrator : Integrator  Orientation=up
  Integrator1 : Integrator  Orientation=up
  Product : Product  SaturateOnIntegerOverflow=on
  Product1 : Product  SaturateOnIntegerOverflow=on
  Product2 : Product  Orientation=left  SaturateOnIntegerOverflow=on
  Product3 : Product  Orientation=left  SaturateOnIntegerOverflow=on
  Sum : Sum  Inputs=|++  SaturateOnIntegerOverflow=on
  Sum1 : Sum  Orientation=up  Inputs=++-  SaturateOnIntegerOverflow=on
  Sum2 : Sum  Orientation=up  Inputs=+|-  SaturateOnIntegerOverflow=on
  Out : Outport
  wires:
  avg_wind/1 -> Coefficients/1(avg_wind)
  Coefficients/4(FD) -> [FD]
  Coefficients/3(ED) -> [ED]
  Coefficients/2(CD) -> [CD]
  Coefficients/1(BD) -> [BD]
  [FD] -> Product3/2
  [ED] -> Product2/2
  [CD] -> Product1/2
  [BD] -> Product/2
  In/1 -> Product1/1, Product/1, A/D/1
  Sum/1 -> Out/1, Product3/1, Product2/1
  Product1/1 -> Sum2/1
  Product3/1 -> Sum2/2
  Sum2/1 -> Integrator1/1
  Product2/1 -> Sum1/3
  Integrator1/1 -> Sum1/2
  Product/1 -> Sum1/1
  Sum1/1 -> Integrator/1
  Integrator/1 -> Sum/2
  A/D/1 -> Sum/1

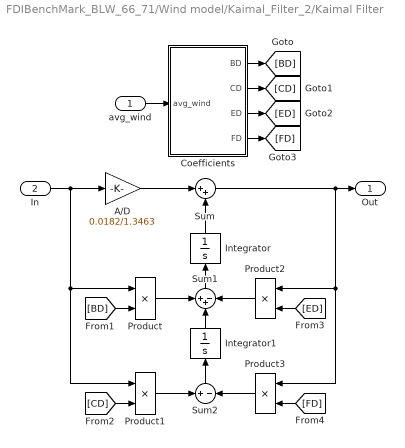
== system FDIBenchMark_BLW_66_71/Wind model/Kaimal_Filter_2/Kaimal Filter ==
  avg_wind : Inport
  In : Inport  Port=2
  A/D : Gain  Gain=0.0182/1.3463  SaturateOnIntegerOverflow=on
  Coefficients : Subsystem
  Integrator : Integrator  Orientation=up
  Integrator1 : Integrator  Orientation=up
  Product : Product  SaturateOnIntegerOverflow=on
  Product1 : Product  SaturateOnIntegerOverflow=on
  Product2 : Product  Orientation=left  SaturateOnIntegerOverflow=on
  Product3 : Product  Orientation=left  SaturateOnIntegerOverflow=on
  Sum : Sum  Inputs=|++  SaturateOnIntegerOverflow=on
  Sum1 : Sum  Orientation=up  Inputs=++-  SaturateOnIntegerOverflow=on
  Sum2 : Sum  Orientation=up  Inputs=+|-  SaturateOnIntegerOverflow=on
  Out : Outport
  wires:
  A/D/1 -> Sum/1
  Integrator/1 -> Sum/2
  Sum1/1 -> Integrator/1
  Product/1 -> Sum1/1
  Integrator1/1 -> Sum1/2
  Product2/1 -> Sum1/3
  Sum2/1 -> Integrator1/1
  Product3/1 -> Sum2/2
  Product1/1 -> Sum2/1
  Sum/1 -> Product2/1, Product3/1, Out/1
  In/1 -> A/D/1, Product/1, Product1/1
  [BD] -> Product/2
  [CD] -> Product1/2
  [ED] -> Product2/2
  [FD] -> Product3/2
  Coefficients/1(BD) -> [BD]
  Coefficients/2(CD) -> [CD]
  Coefficients/3(ED) -> [ED]
  Coefficients/4(FD) -> [FD]
  avg_wind/1 -> Coefficients/1(avg_wind)

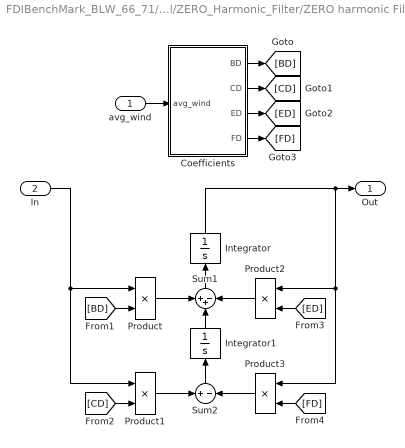
== system FDIBenchMark_BLW_66_71/Wind model/ZERO_Harmonic_Filter/ZERO harmonic Filter ==
  avg_wind : Inport
  In : Inport  Port=2
  Coefficients : Subsystem
  Integrator : Integrator  Orientation=up
  Integrator1 : Integrator  Orientation=up
  Product : Product  SaturateOnIntegerOverflow=on
  Product1 : Product  SaturateOnIntegerOverflow=on
  Product2 : Product  Orientation=left  SaturateOnIntegerOverflow=on
  Product3 : Product  Orientation=left  SaturateOnIntegerOverflow=on
  Sum1 : Sum  Orientation=up  Inputs=++-  SaturateOnIntegerOverflow=on
  Sum2 : Sum  Orientation=up  Inputs=+|-  SaturateOnIntegerOverflow=on
  Out : Outport
  wires:
  Integrator/1 -> Product2/1, Product3/1, Out/1
  Sum1/1 -> Integrator/1
  Product/1 -> Sum1/1
  Integrator1/1 -> Sum1/2
  Product2/1 -> Sum1/3
  Sum2/1 -> Integrator1/1
  Product3/1 -> Sum2/2
  Product1/1 -> Sum2/1
  In/1 -> Product/1, Product1/1
  [BD] -> Product/2
  [CD] -> Product1/2
  [ED] -> Product2/2
  [FD] -> Product3/2
  Coefficients/1(BD) -> [BD]
  Coefficients/2(CD) -> [CD]
  Coefficients/3(ED) -> [ED]
  Coefficients/4(FD) -> [FD]
  avg_wind/1 -> Coefficients/1(avg_wind)

== system FDIBenchMark_BLW_66_71/Wind model/3rd_Harmonic_Filter1/3rd harmonic Filter/Coefficients ==
  avg_wind : Inport
  BD coeff : Fcn  Expr=0.2766/0.3691/(r/u(1))
  CD coeff : Fcn  Expr=0.0307/0.3691/(r/u(1))^2
  ED coeff : Fcn  Expr=1.7722/0.3691/(r/u(1))
  FD coeff : Fcn  Expr=1/0.3691/(r/u(1))^2
  BD : Outport
  CD : Outport  Port=2
  ED : Outport  Port=3
  FD : Outport  Port=4
  wires:
  FD coeff/1 -> FD/1
  ED coeff/1 -> ED/1
  CD coeff/1 -> CD/1
  BD coeff/1 -> BD/1
  avg_wind/1 -> FD coeff/1, ED coeff/1, CD coeff/1, BD coeff/1

== system FDIBenchMark_BLW_66_71/Wind model/Kaimal_Filter_1/Kaimal Filter/Coefficients ==
  avg_wind : Inport
  BD coeff : Fcn  Expr=1.3653/1.3463/(L/2/pi/u(1))
  CD coeff : Fcn  Expr=0.9846/1.3463/(L/2/pi/u(1))^2
  ED coeff : Fcn  Expr=3.7593/1.3463/(L/2/pi/u(1))
  FD coeff : Fcn  Expr=1/1.3463/(L/2/pi/u(1))^2
  BD : Outport
  CD : Outport  Port=2
  ED : Outport  Port=3
  FD : Outport  Port=4
  wires:
  FD coeff/1 -> FD/1
  ED coeff/1 -> ED/1
  CD coeff/1 -> CD/1
  BD coeff/1 -> BD/1
  avg_wind/1 -> FD coeff/1, ED coeff/1, CD coeff/1, BD coeff/1

== system FDIBenchMark_BLW_66_71/Wind model/Kaimal_Filter_2/Kaimal Filter/Coefficients ==
  avg_wind : Inport
  BD coeff : Fcn  Expr=1.3653/1.3463/(L/2/pi/u(1))
  CD coeff : Fcn  Expr=0.9846/1.3463/(L/2/pi/u(1))^2
  ED coeff : Fcn  Expr=3.7593/1.3463/(L/2/pi/u(1))
  FD coeff : Fcn  Expr=1/1.3463/(L/2/pi/u(1))^2
  BD : Outport
  CD : Outport  Port=2
  ED : Outport  Port=3
  FD : Outport  Port=4
  wires:
  avg_wind/1 -> BD coeff/1, CD coeff/1, ED coeff/1, FD coeff/1
  BD coeff/1 -> BD/1
  CD coeff/1 -> CD/1
  ED coeff/1 -> ED/1
  FD coeff/1 -> FD/1

== system FDIBenchMark_BLW_66_71/Wind model/ZERO_Harmonic_Filter/ZERO harmonic Filter/Coefficients ==
  avg_wind : Inport
  BD coeff : Fcn  Expr=4.7869/7.6823/(r/u(1))
  CD coeff : Fcn  Expr=0.9904/7.6823/(r/u(1))^2
  ED coeff : Fcn  Expr=7.3518/7.6823/(r/u(1))
  FD coeff : Fcn  Expr=1/7.6823/(r/u(1))^2
  BD : Outport
  CD : Outport  Port=2
  ED : Outport  Port=3
  FD : Outport  Port=4
  wires:
  avg_wind/1 -> BD coeff/1, CD coeff/1, ED coeff/1, FD coeff/1
  BD coeff/1 -> BD/1
  CD coeff/1 -> CD/1
  ED coeff/1 -> ED/1
  FD coeff/1 -> FD/1

== matlab function Controller/Embedded MATLAB Function ==
  data: P_g input double; ControlZone output double; P_r input double; Omega_g input double; LastControlZone input double; Omega_nom input double; Omega_delta input double
function ControlZone = ZoneControl(P_g, P_r, Omega_g, LastControlZone,Omega_nom,Omega_delta)
 
if LastControlZone==0,
    if (P_g>=P_r) ||(Omega_g>=Omega_nom)
        ControlZone=1;
    else
        ControlZone=0;
    end
else
    if (Omega_g<(Omega_nom-Omega_delta))
        ControlZone=0;
    else
        ControlZone=1;
    end
end
